simulink model "Quiz4_PartC"  (R2017b)
settings: Solver=VariableStepAuto  StartTime=0.0  StopTime=10.0  RelTol=1e-3
undefined symbols (not defined in the file): b, w, Z
libraries: fl_lib x5, sdl_lib x1
settings Model: Creator=Harrison  LastModifiedBy=Harrison

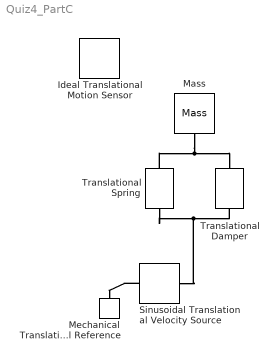
== system Quiz4_PartC ==
  Ideal Translational Motion Sensor : fl_lib/Mechanical/Mechanical Sensors/Ideal Translational Motion Sensor  offset=0 m
  Mass : fl_lib/Mechanical/Translational Elements/Mass  mass=m kg  v_specify=off  v_priority=High  v=0 m/s  v_nominal_specify=off  v_nominal_unit=m/s  v_nominal_value=1  f_specify=off  f_priority=None  f=0 N  f_nominal_specify=off  f_nominal_unit=N  f_nominal_value=1
  Mechanical Translational Reference : fl_lib/Mechanical/Translational Elements/Mechanical Translational Reference
  Sinusoidal Translational Velocity Source : sdl_lib/Sources/Sinusoidal Translational Velocity Source  offset=0 m/s  amplitude=Z*w m/s  phase_shift=pi/2 rad  frequency=w/(2*pi) Hz
      settings: SourceProductName=Simscape Driveline  SourceProductBaseCode=LD
  Translational Damper : fl_lib/Mechanical/Translational Elements/Translational Damper  D=b N/(m/s)  v_specify=off  v_priority=None  v=0 m/s  v_nominal_specify=off  v_nominal_unit=m/s  v_nominal_value=1  f_specify=off  f_priority=None  f=0 N  f_nominal_specify=off  f_nominal_unit=N  f_nominal_value=1
  Translational Spring : fl_lib/Mechanical/Translational Elements/Translational Spring  spr_rate=k N/m  v_specify=off  v_priority=None  v=0 m/s  v_nominal_specify=off  v_nominal_unit=m/s  v_nominal_value=1  f_specify=off  f_priority=None  f=0 N  f_nominal_specify=off  f_nominal_unit=N  f_nominal_value=1  x_specify=off  x_priority=High  x=0 m  x_nominal_specify=off  x_nominal_unit=m  x_nominal_value=1
  connections:
  Translational Spring/LConn1 -- Mass/LConn1 -- Translational Damper/LConn1
  Translational Spring/RConn1 -- Sinusoidal Translational Velocity Source/RConn1 -- Translational Damper/RConn1
  Sinusoidal Translational Velocity Source/LConn1 -- Mechanical Translational Reference/LConn1
